simulink library "model_lib"  (Simulink 6.3)
undefined symbols (not defined in the file or in its folder): ADQUANT, alt_alp, alt_delt, alt_gamma, alt_ht, alt_R, alt_T0, atmos, att_trim_IC, constants, dc_L2W_IC, DiscIntNeverNeededParam, dtsim, enforce_fuel, inertia_maxprop, inertia_noprop, latlonh_IC, MACH, MACH_att_int_IC, MACH_att_Kb, MACH_att_Kc, MACH_att_Ki, MACH_pos_IC, MACH_pos_int_IC, MACH_pos_Kb, MACH_pos_Kc, MACH_pos_Ki, MACH_pqr_IC, MACH_pqr_int_IC, MACH_pqr_Kb, MACH_pqr_Kc, MACH_pqr_Ki, MACH_quat_IC, MACH_vel_IC, MACH_vel_int_IC, MACH_vel_Kb, MACH_vel_Kc, MACH_vel_Ki, mass_maxprop, mass_noprop, obac_params, r_accel, r_cg_maxprop, r_cg_noprop, r_prop, rho_sl, SENS, SERVO, throttle_idx, tvc_idx, use_NdEdh_pos, use_wind_meas_sim, use_xdot_ground, vehicle_params
libraries: utility_lib x22, model_lib x18, simulink x14, aerospace x1
(part 2 of 2)

== system model_lib/ideal responses/ideal pos vel response ==
  note: Note: If pos cv is is shifted to zero, add pos_IC after feedback pickoff.
      | If pos cv is real position values, set integrator IC to pos_IC
  control_input : Inport
  Constant4 : Constant  Value=MACH_pos_IC*0
  Discrete-Time Integrator1 : DiscreteIntegrator  InitialCondition=MACH_vel_IC  SampleTime=-1  ICPrevOutput=DiscIntNeverNeededParam  ICPrevScaledInput=DiscIntNeverNeededParam
  Discrete-Time Integrator3 : DiscreteIntegrator  InitialCondition=MACH_pos_IC  SampleTime=-1  ICPrevOutput=DiscIntNeverNeededParam  ICPrevScaledInput=DiscIntNeverNeededParam
  Mux : Mux  Inputs=2
  Mux1 : Mux  Inputs=2
  Selector2 : Selector  ElementSrc=External  Elements=[4 5 3]  InputPortWidth=6
  Selector3 : Selector  ElementSrc=External  Elements=[1 2 6]  InputPortWidth=6
  Sum1 : Sum  Inputs=++|  SaturateOnIntegerOverflow=on  InputSameDT=on
  To Workspace : ToWorkspace  VariableName=ideal_pos  SampleTime=MACH.dt  SaveFormat=Array
  To Workspace1 : ToWorkspace  VariableName=ideal_vel  SampleTime=MACH.dt  SaveFormat=Array
  get posvel cmd : Subsystem
  pos loop : Subsystem
  vel loop : Subsystem
  wires:
  Discrete-Time Integrator3/1 -> Sum1/2, pos loop/2(NEh), Mux/2
  Mux/1 -> Selector2/1
  vel loop/1(NEhdotdot) -> Discrete-Time Integrator1/1
  Sum1/1 -> To Workspace/1
  Constant4/1 -> Sum1/1
  Selector3/1 -> vel loop/1(NEhdot_cmd)
  pos loop/1(NEhdot_cmd) -> Mux1/2
  get posvel cmd/1(posvel_cmd) -> Mux/1, Mux1/1  "NEh"
  Mux1/1 -> Selector3/1
  control_input/1 -> get posvel cmd/1(control_input)
  get posvel cmd/3(vel_select) -> Selector3/2
  get posvel cmd/2(pos_select) -> Selector2/2
  Selector2/1 -> pos loop/1(NEh_cmd)
  Discrete-Time Integrator1/1 -> Discrete-Time Integrator3/1, To Workspace1/1, vel loop/2(NEhdot)

== system model_lib/mkplt output/angles ==
  dircos : Inport
  uvw : Inport  Port=2
  NED_wind : Inport  Port=3
  dc2mba : utility_lib/dc2mba
  dc2tiltcam : utility_lib/dc2tiltcam
  dc2ypr : utility_lib/dc2ypr
  relative wind velocity : model_lib/relative wind velocity
  uvw_rw : Outport
  tilta;tiltb;cam : Outport  Port=2
  phi;theta;psi : Outport  Port=3
  mu;alpha;beta : Outport  Port=4
  wires:
  NED_wind/1 -> relative wind velocity/3
  uvw/1 -> relative wind velocity/1
  dircos/1 -> relative wind velocity/2, dc2mba/1, dc2tiltcam/1, dc2ypr/1
  dc2mba/1 -> mu;alpha;beta/1
  dc2tiltcam/1 -> tilta;tiltb;cam/1
  dc2ypr/1 -> phi;theta;psi/1
  relative wind velocity/1 -> uvw_rw/1

== system model_lib/model accels/accel at cg ==
  uvw_dot : Inport
  gvec : Inport  Port=2
  uvw : Inport  Port=3
  pqr : Inport  Port=4
  Sum10 : Sum  Inputs=++-  SaturateOnIntegerOverflow=on  InputSameDT=on
  omega x Vb : utility_lib/cross product
  a_cg : Outport
  wires:
  gvec/1 -> Sum10/3
  pqr/1 -> omega x Vb/1
  uvw/1 -> omega x Vb/2
  Sum10/1 -> a_cg/1
  omega x Vb/1 -> Sum10/2
  uvw_dot/1 -> Sum10/1

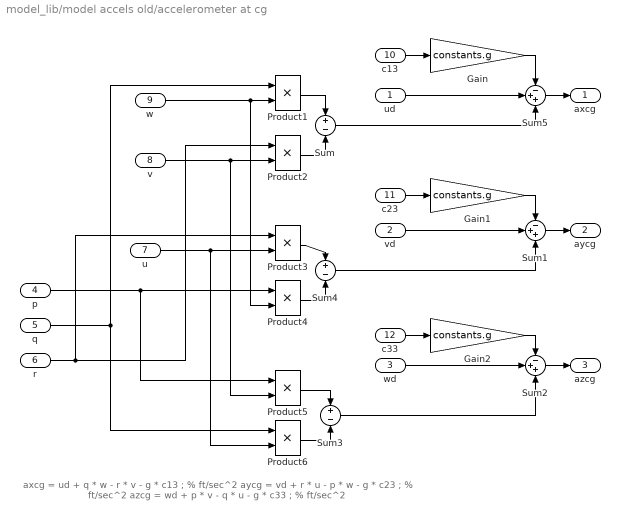
== system model_lib/model accels old/accelerometer at cg ==
  note: axcg =  ud + q * w - r * v - g * c13 ; % ft/sec^2
      | aycg =  vd + r * u - p * w - g * c23 ; % ft/sec^2
      | azcg =  wd + p * v - q * u - g * c33 ; % ft/sec^2
  ud : Inport
  vd : Inport  Port=2
  wd : Inport  Port=3
  p : Inport  Port=4
  q : Inport  Port=5
  r : Inport  Port=6
  u : Inport  Port=7
  v : Inport  Port=8
  w : Inport  Port=9
  c13 : Inport  Port=10
  c23 : Inport  Port=11
  c33 : Inport  Port=12
  Gain : Gain  Gain=constants.g  SaturateOnIntegerOverflow=on
  Gain1 : Gain  Gain=constants.g  SaturateOnIntegerOverflow=on
  Gain2 : Gain  Gain=constants.g  SaturateOnIntegerOverflow=on
  Product{1..6} (6 alike) : Product  SaturateOnIntegerOverflow=on
  Sum : Sum  Inputs=+-  SaturateOnIntegerOverflow=on  InputSameDT=on
  Sum1 : Sum  Inputs=-++  SaturateOnIntegerOverflow=on  InputSameDT=on
  Sum2 : Sum  Inputs=-++  SaturateOnIntegerOverflow=on  InputSameDT=on
  Sum3 : Sum  Inputs=+-  SaturateOnIntegerOverflow=on  InputSameDT=on
  Sum4 : Sum  Inputs=+-  SaturateOnIntegerOverflow=on  InputSameDT=on
  Sum5 : Sum  Inputs=-++  SaturateOnIntegerOverflow=on  InputSameDT=on
  axcg : Outport
  aycg : Outport  Port=2
  azcg : Outport  Port=3
  wires:
  Sum5/1 -> axcg/1
  ud/1 -> Sum5/2
  vd/1 -> Sum1/2
  Sum1/1 -> aycg/1
  wd/1 -> Sum2/2
  Sum2/1 -> azcg/1
  q/1 -> Product1/1, Product6/1
  w/1 -> Product1/2, Product4/2
  Product1/1 -> Sum/1
  v/1 -> Product2/2, Product5/2
  r/1 -> Product2/1, Product3/1
  Product2/1 -> Sum/2
  Sum/1 -> Sum5/3
  c13/1 -> Gain/1
  Gain/1 -> Sum5/1
  c23/1 -> Gain1/1
  Gain1/1 -> Sum1/1
  c33/1 -> Gain2/1
  Gain2/1 -> Sum2/1
  u/1 -> Product3/2, Product6/2
  p/1 -> Product4/1, Product5/1
  Product4/1 -> Sum4/2
  Product3/1 -> Sum4/1
  Product5/1 -> Sum3/1
  Product6/1 -> Sum3/2
  Sum3/1 -> Sum2/3
  Sum4/1 -> Sum1/3

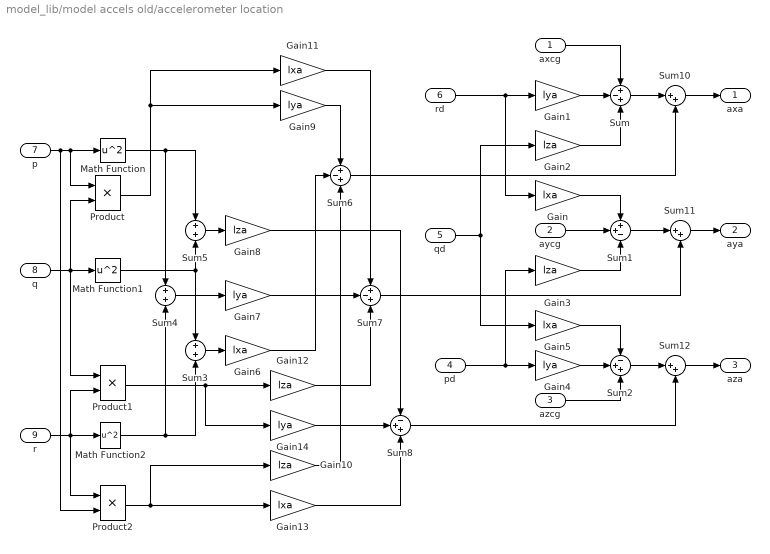
== system model_lib/model accels old/accelerometer location ==
  axcg : Inport
  aycg : Inport  Port=2
  azcg : Inport  Port=3
  pd : Inport  Port=4
  qd : Inport  Port=5
  rd : Inport  Port=6
  p : Inport  Port=7
  q : Inport  Port=8
  r : Inport  Port=9
  Gain{,5..6,11,13} (5 alike) : Gain  Gain=lxa  SaturateOnIntegerOverflow=on
  Gain{1,4,7,9,14} (5 alike) : Gain  Gain=lya  SaturateOnIntegerOverflow=on
  Gain{2..3,8,10,12} (5 alike) : Gain  Gain=lza  SaturateOnIntegerOverflow=on
  Math Function : Math  Operator=square  SaturateOnIntegerOverflow=on
  Math Function1 : Math  Operator=square  SaturateOnIntegerOverflow=on
  Math Function2 : Math  Operator=square  SaturateOnIntegerOverflow=on
  Product : Product  SaturateOnIntegerOverflow=on
  Product1 : Product  SaturateOnIntegerOverflow=on
  Product2 : Product  SaturateOnIntegerOverflow=on
  Sum : Sum  Inputs=+-+  SaturateOnIntegerOverflow=on  InputSameDT=on
  Sum1 : Sum  Inputs=++-  SaturateOnIntegerOverflow=on  InputSameDT=on
  Sum10 : Sum  Inputs=|++  SaturateOnIntegerOverflow=on  InputSameDT=on
  Sum11 : Sum  Inputs=|++  SaturateOnIntegerOverflow=on  InputSameDT=on
  Sum12 : Sum  Inputs=|++  SaturateOnIntegerOverflow=on  InputSameDT=on
  Sum2 : Sum  Inputs=-++  SaturateOnIntegerOverflow=on  InputSameDT=on
  Sum3 : Sum  SaturateOnIntegerOverflow=on  InputSameDT=on
  Sum4 : Sum  SaturateOnIntegerOverflow=on  InputSameDT=on
  Sum5 : Sum  SaturateOnIntegerOverflow=on  InputSameDT=on
  Sum6 : Sum  Inputs=+-+  SaturateOnIntegerOverflow=on  InputSameDT=on
  Sum7 : Sum  Inputs=+-+  SaturateOnIntegerOverflow=on  InputSameDT=on
  Sum8 : Sum  Inputs=-++  SaturateOnIntegerOverflow=on  InputSameDT=on
  axa : Outport
  aya : Outport  Port=2
  aza : Outport  Port=3
  wires:
  axcg/1 -> Sum/1
  aycg/1 -> Sum1/2
  azcg/1 -> Sum2/3
  Gain1/1 -> Sum/2
  Gain2/1 -> Sum/3
  qd/1 -> Gain2/1, Gain5/1
  rd/1 -> Gain1/1, Gain/1
  Gain3/1 -> Sum1/3
  Gain/1 -> Sum1/1
  pd/1 -> Gain3/1, Gain4/1
  Gain4/1 -> Sum2/2
  Gain5/1 -> Sum2/1
  p/1 -> Product/1, Math Function/1, Product2/2
  r/1 -> Math Function2/1, Product1/2, Product2/1
  q/1 -> Math Function1/1, Product/2, Product1/1
  Math Function/1 -> Sum4/1, Sum5/1
  Math Function1/1 -> Sum3/1, Sum5/2
  Math Function2/1 -> Sum3/2, Sum4/2
  Sum3/1 -> Gain6/1
  Sum4/1 -> Gain7/1
  Sum5/1 -> Gain8/1
  Product/1 -> Gain9/1, Gain11/1
  Product2/1 -> Gain10/1, Gain13/1
  Product1/1 -> Gain12/1, Gain14/1
  Gain6/1 -> Sum6/2
  Gain9/1 -> Sum6/1
  Gain10/1 -> Sum6/3
  Gain7/1 -> Sum7/2
  Gain11/1 -> Sum7/1
  Gain12/1 -> Sum7/3
  Gain8/1 -> Sum8/1
  Gain13/1 -> Sum8/3
  Gain14/1 -> Sum8/2
  Sum/1 -> Sum10/1
  Sum10/1 -> axa/1
  Sum1/1 -> Sum11/1
  Sum11/1 -> aya/1
  Sum2/1 -> Sum12/1
  Sum12/1 -> aza/1
  Sum6/1 -> Sum10/2
  Sum7/1 -> Sum11/2
  Sum8/1 -> Sum12/2

== system model_lib/Sensor Errors/Sensor Errors/Sensor Model  ==
  note: Sensor Model
  y : Inport
  Band-Limited White Noise1 : simulink/Sources/Band-Limited White Noise  Cov=ones(1,SENS.nsens)  Ts=dtsim  seed=SENS.seed
  Bias : Constant  Value=SENS.bias
  Drift : simulink/Sources/Ramp  slope=SENS.drift  start=0  X0=0
  Integrator : Integrator
  SQRT(2*beta) : Gain  Gain="sqrt(2.0  .*  SENS.beta)"  SaturateOnIntegerOverflow=on
  Sum : Sum  Inputs=|++  SampleTime=dtsim  SaturateOnIntegerOverflow=on  InputSameDT=on
  Sum1 : Sum  Inputs=|+-  SaturateOnIntegerOverflow=on  InputSameDT=on
  Sum2 : Sum  Orientation=up  Inputs=++|  SaturateOnIntegerOverflow=on  InputSameDT=on
  Sum3 : Sum  Orientation=up  Inputs=++|  SaturateOnIntegerOverflow=on  InputSameDT=on
  beta : Gain  Orientation=left  Gain=SENS.beta  SaturateOnIntegerOverflow=on
  sigma : Gain  Gain=SENS.sig  SaturateOnIntegerOverflow=on
  y_sens : Outport
  wires:
  y/1 -> Sum/1
  Drift/1 -> Sum3/2
  Bias/1 -> Sum3/1
  Sum3/1 -> Sum2/2
  Integrator/1 -> beta/1, Sum2/1
  Sum1/1 -> Integrator/1
  beta/1 -> Sum1/2
  SQRT(2*beta)/1 -> Sum1/1
  sigma/1 -> SQRT(2*beta)/1
  Sum2/1 -> Sum/2
  Sum/1 -> y_sens/1
  Band-Limited White Noise1/1 -> sigma/1

== system model_lib/Sensor Errors/Sensor Errors/normalize quaternions ==
  y_sens_in : Inport
  Assignment : Assignment  Elements=SENS.quat_idx
  Dot Product : simulink/Math Operations/Dot Product  InputSameDT=on  OutDataType=sfix(16)  OutScaling=2^-10  DoSatur=off
  Math Function1 : Math  Operator=sqrt  SaturateOnIntegerOverflow=on
  Product : Product  Inputs=*/  SaturateOnIntegerOverflow=on
  Selector : Selector  Elements=SENS.quat_idx  InputPortWidth=SENS.nsens
  y_sens_out : Outport
  wires:
  Math Function1/1 -> Product/2
  Selector/1 -> Product/1, Dot Product/1, Dot Product/2
  Product/1 -> Assignment/2
  y_sens_in/1 -> Selector/1, Assignment/1
  Assignment/1 -> y_sens_out/1
  Dot Product/1 -> Math Function1/1

== system model_lib/get atmos_env/air density/stratosphere ==
  h : Inport
  Constant : Constant  Value=alt_alp
  Constant1 : Constant  Value=alt_R
  Constant2 : Constant  Value=alt_T0
  Constant4 : Constant  Value=alt_ht
  Math Function : Math  SaturateOnIntegerOverflow=on
  Product1 : Product  Inputs=**  RndMeth=Zero
  Product2 : Product  Inputs=*//  RndMeth=Zero
  Product3 : Product  Inputs=/*  RndMeth=Zero
  Product4 : Product  Inputs=/**  RndMeth=Zero
  Sum2 : Sum  Inputs=-+|
  Sum3 : Sum  Inputs=|+-
  alt_prt : Constant  Value=alt_delt
  sig : Outport
  wires:
  Constant2/1 -> Sum2/2, Product3/2
  Product1/1 -> Sum2/1
  h/1 -> Sum3/1
  Constant4/1 -> Sum3/2, Product1/1
  Constant/1 -> Product1/2
  Sum3/1 -> Product2/1
  Sum2/1 -> Product2/3, Product3/1
  Constant1/1 -> Product2/2
  Product2/1 -> Math Function/1
  Math Function/1 -> Product4/1
  Product3/1 -> Product4/2
  Product4/1 -> sig/1
  alt_prt/1 -> Product4/3

== system model_lib/get atmos_env/air density/troposphere ==
  h : Inport
  Constant : Constant  Value=alt_alp
  Constant1 : Constant  Value=alt_R
  Constant2 : Constant  Value=alt_T0
  Constant3 : Constant
  Constant4 : Constant
  Math Function : Math  Operator=pow  SaturateOnIntegerOverflow=on
  Product : Product  Inputs=*/*  RndMeth=Zero
  Product1 : Product  Inputs=//  RndMeth=Zero
  Sum1 : Sum  Inputs=|+-
  Sum2 : Sum  Inputs=-+|
  sig : Outport
  wires:
  h/1 -> Product/1
  Constant3/1 -> Sum1/1
  Product/1 -> Sum1/2
  Constant2/1 -> Product/2
  Constant/1 -> Product/3, Product1/1
  Constant1/1 -> Product1/2
  Product1/1 -> Sum2/2
  Constant4/1 -> Sum2/1
  Sum1/1 -> Math Function/1
  Sum2/1 -> Math Function/2
  Math Function/1 -> sig/1

== system model_lib/get atmos_env/air temp/stratosphere ==
  Constant : Constant  Value=alt_alp
  Constant2 : Constant  Value=alt_T0
  Constant4 : Constant  Value=alt_ht
  Product1 : Product  Inputs=**  RndMeth=Zero
  Sum2 : Sum  Inputs=-+|
  T : Outport
  wires:
  Sum2/1 -> T/1
  Constant/1 -> Product1/2
  Constant4/1 -> Product1/1
  Product1/1 -> Sum2/1
  Constant2/1 -> Sum2/2

== system model_lib/get atmos_env/air temp/troposphere ==
  h : Inport
  Constant5 : Constant  Value=alt_alp
  Constant6 : Constant  Value=alt_T0
  Product2 : Product  Inputs=**  RndMeth=Zero
  Sum3 : Sum  Inputs=-+|
  T : Outport
  wires:
  Sum3/1 -> T/1
  Constant5/1 -> Product2/2
  h/1 -> Product2/1
  Product2/1 -> Sum3/1
  Constant6/1 -> Sum3/2

== system model_lib/ideal responses/ideal att rate response/att loop ==
  e_cmd : Inport
  e : Inport  Port=2
  Discrete-Time Integrator : DiscreteIntegrator  IntegratorMethod=Integration: Backward Euler  InitialCondition=MACH_att_int_IC  SampleTime=-1  ICPrevOutput=DiscIntNeverNeededParam  ICPrevScaledInput=DiscIntNeverNeededParam
  Gain1 : Gain  Gain=MACH_att_Kb  SaturateOnIntegerOverflow=on
  Gain4 : Gain  Gain=MACH_att_Kc  SaturateOnIntegerOverflow=on
  Gain5 : Gain  Gain=MACH_att_Ki.*MACH_att_Kb  SaturateOnIntegerOverflow=on
  Sum2 : Sum  Inputs=|+-  SaturateOnIntegerOverflow=on  InputSameDT=on
  Sum3 : Sum  Inputs=++-  SaturateOnIntegerOverflow=on  InputSameDT=on
  Terminator : Terminator
  getedinv : utility_lib/getedinv
  pqr_cmd : Outport
  wires:
  Gain1/1 -> getedinv/1
  Gain5/1 -> Discrete-Time Integrator/1
  Discrete-Time Integrator/1 -> Sum3/2
  Gain4/1 -> Sum3/1
  Sum3/1 -> Gain1/1
  Sum2/1 -> Gain5/1
  e_cmd/1 -> Sum2/1, Gain4/1
  getedinv/1 -> pqr_cmd/1
  e/1 -> Sum2/2, Sum3/3, getedinv/2
  getedinv/2 -> Terminator/1

== system model_lib/ideal responses/ideal att rate response/get att cmd ==
  note: Note: So that we can switch between a pqr command
      | and a quat command, the 4th component of command (throt)
      | is left until after the switch, and removed later.
  control_input : Inport
  e : Inport  Port=2
  Bus Selector1 : BusSelector  OutputSignals=mode_sw.CLAW_mode,command
  Constant1 : Constant  Value=[0 0 0 0]
  Constant2 : Constant  Value=[5 6 7 8]
  Constant3 : Constant  Value=[4 5 6]
  Constant4 : Constant  Value=[1 2 3]
  Constant5 : Constant  Value=[1 2 3 4]
  Multiport Switch1 : MultiPortSwitch  Inputs=6  zeroidx=on
  Multiport Switch2 : MultiPortSwitch  Inputs=6  zeroidx=on
  Multiport Switch3 : MultiPortSwitch  Inputs=6  zeroidx=on
  convert to quat : Subsystem
  quatpqr_cmd : Outport
  quat_select : Outport  Port=2
  pqr_select : Outport  Port=3
  wires:
  control_input/1 -> Bus Selector1/1
  Multiport Switch1/1 -> quatpqr_cmd/1
  Bus Selector1/1 -> Multiport Switch1/1, Multiport Switch2/1, Multiport Switch3/1  "<CLAW_mode>"
  Constant1/1 -> Multiport Switch1/2, Multiport Switch1/5, Multiport Switch1/6, Multiport Switch1/7
  Multiport Switch2/1 -> quat_select/1
  Multiport Switch3/1 -> pqr_select/1
  Constant2/1 -> Multiport Switch2/2, Multiport Switch2/3, Multiport Switch2/5, Multiport Switch2/6, Multiport Switch2/7
  Constant3/1 -> Multiport Switch3/2, Multiport Switch3/4, Multiport Switch3/5, Multiport Switch3/6, Multiport Switch3/7
  Bus Selector1/2 -> Multiport Switch1/3, convert to quat/1(att_cmd)  "<command>"
  Constant5/1 -> Multiport Switch2/4
  convert to quat/1(e_cmd) -> Multiport Switch1/4
  Constant4/1 -> Multiport Switch3/3
  e/1 -> convert to quat/2(e)

== system model_lib/ideal responses/ideal att rate response/rate loop ==
  pqr_cmd : Inport
  pqr : Inport  Port=2
  Discrete-Time Integrator : DiscreteIntegrator  IntegratorMethod=Integration: Backward Euler  InitialCondition=MACH_pqr_int_IC  SampleTime=-1  ICPrevOutput=DiscIntNeverNeededParam  ICPrevScaledInput=DiscIntNeverNeededParam
  Gain : Gain  Gain=MACH_pqr_Kb  SaturateOnIntegerOverflow=on
  Gain2 : Gain  Gain=MACH_pqr_Kc  SaturateOnIntegerOverflow=on
  Gain3 : Gain  Gain=MACH_pqr_Ki.*MACH_pqr_Kb  SaturateOnIntegerOverflow=on
  Sum : Sum  Inputs=|+-  SaturateOnIntegerOverflow=on  InputSameDT=on
  Sum1 : Sum  Inputs=++-  SaturateOnIntegerOverflow=on  InputSameDT=on
  pqrdot : Outport
  wires:
  Sum/1 -> Gain3/1
  pqr_cmd/1 -> Gain2/1, Sum/1
  Gain/1 -> pqrdot/1
  Sum1/1 -> Gain/1
  Gain2/1 -> Sum1/1
  Discrete-Time Integrator/1 -> Sum1/2
  Gain3/1 -> Discrete-Time Integrator/1
  pqr/1 -> Sum/2, Sum1/3

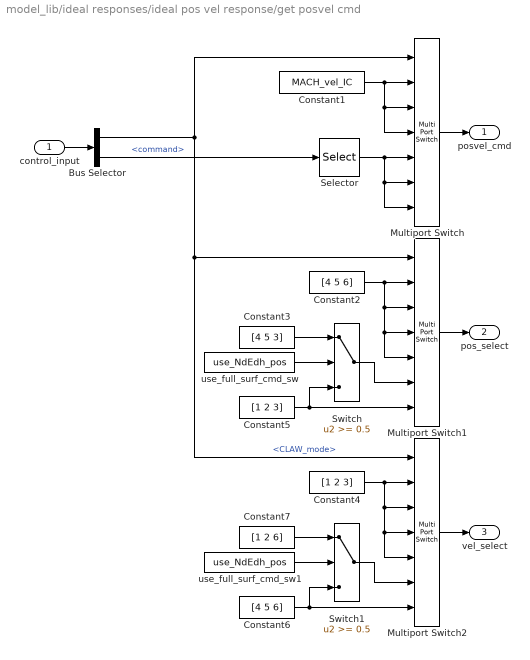
== system model_lib/ideal responses/ideal pos vel response/get posvel cmd ==
  control_input : Inport
  Bus Selector : BusSelector  OutputSignals=mode_sw.CLAW_mode,command
  Constant1 : Constant  Value=MACH_vel_IC
  Constant2 : Constant  Value=[4 5 6]
  Constant3 : Constant  Value=[4 5 3]
  Constant4 : Constant  Value=[1 2 3]
  Constant5 : Constant  Value=[1 2 3]
  Constant6 : Constant  Value=[4 5 6]
  Constant7 : Constant  Value=[1 2 6]
  Multiport Switch : MultiPortSwitch  Inputs=6  zeroidx=on
  Multiport Switch1 : MultiPortSwitch  Inputs=6  zeroidx=on
  Multiport Switch2 : MultiPortSwitch  Inputs=6  zeroidx=on
  Selector : Selector  Elements=[1 2 4]  InputPortWidth=4
  Switch : Switch  Threshold=0.5
  Switch1 : Switch  Threshold=0.5
  use_full_surf_cmd_sw : Constant  Value=use_NdEdh_pos
  use_full_surf_cmd_sw1 : Constant  Value=use_NdEdh_pos
  posvel_cmd : Outport
  pos_select : Outport  Port=2
  vel_select : Outport  Port=3
  wires:
  Multiport Switch/1 -> posvel_cmd/1
  Bus Selector/1 -> Multiport Switch/1, Multiport Switch1/1, Multiport Switch2/1  "<CLAW_mode>"
  control_input/1 -> Bus Selector/1
  Constant1/1 -> Multiport Switch/2, Multiport Switch/3, Multiport Switch/4
  Selector/1 -> Multiport Switch/5, Multiport Switch/6, Multiport Switch/7
  Multiport Switch1/1 -> pos_select/1
  Multiport Switch2/1 -> vel_select/1
  Constant2/1 -> Multiport Switch1/2, Multiport Switch1/3, Multiport Switch1/4, Multiport Switch1/5
  Switch/1 -> Multiport Switch1/6
  Constant4/1 -> Multiport Switch2/2, Multiport Switch2/3, Multiport Switch2/4, Multiport Switch2/5
  Constant5/1 -> Multiport Switch1/7, Switch/3
  Constant6/1 -> Multiport Switch2/7, Switch1/3
  Switch1/1 -> Multiport Switch2/6
  Bus Selector/2 -> Selector/1  "<command>"
  use_full_surf_cmd_sw/1 -> Switch/2
  Constant3/1 -> Switch/1
  Constant7/1 -> Switch1/1
  use_full_surf_cmd_sw1/1 -> Switch1/2

== system model_lib/ideal responses/ideal pos vel response/pos loop ==
  NEh_cmd : Inport
  NEh : Inport  Port=2
  Discrete-Time Integrator : DiscreteIntegrator  IntegratorMethod=Integration: Backward Euler  InitialCondition=MACH_pos_int_IC  SampleTime=-1  ICPrevOutput=DiscIntNeverNeededParam  ICPrevScaledInput=DiscIntNeverNeededParam
  Gain1 : Gain  Gain=MACH_pos_Kb  SaturateOnIntegerOverflow=on
  Gain4 : Gain  Gain=MACH_pos_Kc  SaturateOnIntegerOverflow=on
  Gain5 : Gain  Gain=MACH_pos_Ki.*MACH_pos_Kb  SaturateOnIntegerOverflow=on
  Sum2 : Sum  Inputs=|+-  SaturateOnIntegerOverflow=on  InputSameDT=on
  Sum3 : Sum  Inputs=++-  SaturateOnIntegerOverflow=on  InputSameDT=on
  NEhdot_cmd : Outport
  wires:
  Sum2/1 -> Gain5/1
  Sum3/1 -> Gain1/1
  Gain4/1 -> Sum3/1
  Discrete-Time Integrator/1 -> Sum3/2
  Gain5/1 -> Discrete-Time Integrator/1
  Gain1/1 -> NEhdot_cmd/1
  NEh_cmd/1 -> Sum2/1, Gain4/1
  NEh/1 -> Sum2/2, Sum3/3

== system model_lib/ideal responses/ideal pos vel response/vel loop ==
  NEhdot_cmd : Inport
  NEhdot : Inport  Port=2
  Discrete-Time Integrator1 : DiscreteIntegrator  IntegratorMethod=Integration: Backward Euler  InitialCondition=MACH_vel_int_IC  SampleTime=-1  ICPrevOutput=DiscIntNeverNeededParam  ICPrevScaledInput=DiscIntNeverNeededParam
  Gain : Gain  Gain=MACH_vel_Kb  SaturateOnIntegerOverflow=on
  Gain2 : Gain  Gain=MACH_vel_Kc  SaturateOnIntegerOverflow=on
  Gain3 : Gain  Gain=MACH_vel_Ki.*MACH_vel_Kb  SaturateOnIntegerOverflow=on
  Sum : Sum  Inputs=|+-  SaturateOnIntegerOverflow=on  InputSameDT=on
  Sum1 : Sum  Inputs=++-  SaturateOnIntegerOverflow=on  InputSameDT=on
  NEhdotdot : Outport
  wires:
  Sum/1 -> Gain3/1
  NEhdot_cmd/1 -> Gain2/1, Sum/1
  Gain/1 -> NEhdotdot/1
  Sum1/1 -> Gain/1
  Gain2/1 -> Sum1/1
  Discrete-Time Integrator1/1 -> Sum1/2
  Gain3/1 -> Discrete-Time Integrator1/1
  NEhdot/1 -> Sum/2, Sum1/3

== system model_lib/ideal responses/ideal att rate response/get att cmd/convert to quat ==
  att_cmd : Inport
  e : Inport  Port=2
  Demux : Demux  Outputs=[2 1]
  Discrete-Time Integrator4 : DiscreteIntegrator  IntegratorMethod=Integration: Backward Euler  InitialCondition=att_trim_IC(3)  SampleTime=-1  ICPrevOutput=DiscIntNeverNeededParam  ICPrevScaledInput=DiscIntNeverNeededParam
  From Workspace2 : FromWorkspace  VariableName=use_cam_rate_cmd_fw  SampleTime=MACH.dt  Interpolate=off  OutputAfterFinalValue=Holding final value
  Multiport Switch1 : MultiPortSwitch  Inputs=2  zeroidx=on
  Mux2 : Mux  Inputs=2
  Selector : Selector  Elements=[1 2 3]  InputPortWidth=4
  att2dc : utility_lib/att2dc
  dc2e_ref : utility_lib/dc2e_ref
  e_cmd : Outport
  wires:
  From Workspace2/1 -> Multiport Switch1/1
  Discrete-Time Integrator4/1 -> Multiport Switch1/3
  Demux/2 -> Multiport Switch1/2, Discrete-Time Integrator4/1
  Multiport Switch1/1 -> Mux2/2
  Demux/1 -> Mux2/1
  att_cmd/1 -> Selector/1
  Selector/1 -> Demux/1
  att2dc/1 -> dc2e_ref/1
  e/1 -> dc2e_ref/2
  Mux2/1 -> att2dc/1
  dc2e_ref/1 -> e_cmd/1
